simulink model "test_simulink"  (R2019b)
settings: Solver=ode45  StartTime=0.0  StopTime=10  RelTol=1e-3
settings Model: Creator=bitgar  LastModifiedBy=zczhu

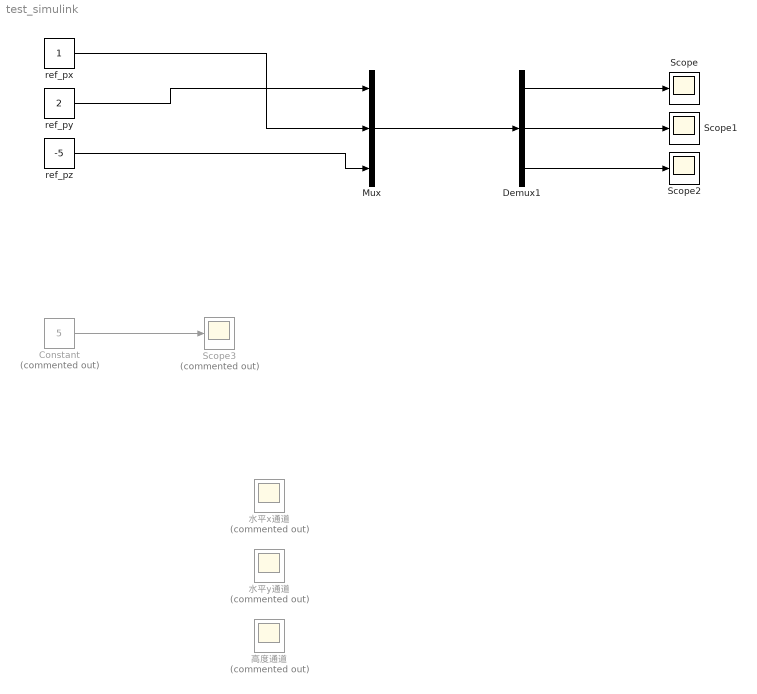
== system test_simulink ==
  Constant : Constant  Commented=on  Value=5  SampleTime=-1
  Demux1 : Demux  Outputs=3
  Mux : Mux  Inputs=3
  Scope : Scope
  Scope1 : Scope
  Scope2 : Scope
  Scope3 : Scope  Commented=on
  ref_px : Constant  SampleTime=-1
  ref_py : Constant  Value=2  SampleTime=-1
  ref_pz : Constant  Value=-5  SampleTime=-1
  水平x通道 : Scope  Commented=on  NumInputPorts=2
  水平y通道 : Scope  Commented=on  NumInputPorts=2
  高度通道 : Scope  Commented=on  NumInputPorts=2
  wires:
  ref_px/1 -> Mux/2
  ref_py/1 -> Mux/1
  ref_pz/1 -> Mux/3
  Mux/1 -> Demux1/1
  Constant/1 -> Scope3/1
  Demux1/1 -> Scope/1
  Demux1/2 -> Scope1/1
  Demux1/3 -> Scope2/1
